simulink model "exampleModel_bus_axi_w_4ptavg"  (R2017b)
settings: Solver=VariableStepAuto  StartTime=0.0  StopTime=10e-5  RelTol=1e-3
PreLoadFcn:
  | setup
values from neighbouring files (symbols this model uses):
  axiClk = 156.25e6    (= 156250000)    [setup.m]    (also in setup_exampleModel_bus_axi_simulink.m; setup_exampleModel_bus_axi_simulink_lcls2.m; setup_lcls2_pcav.m; sysgen_signal.m)
  cav1p1_addr = 204    [setup_exampleModel_bus_axi_simulink.m]    (also in setup_exampleModel_bus_axi_simulink_lcls2.m; setup_lcls2_pcav.m; sysgen_signal.m)
  cav1p2_addr = cav1p1_addr * 2    (= 408)    [setup_exampleModel_bus_axi_simulink.m]    (also in setup_exampleModel_bus_axi_simulink_lcls2.m; setup_lcls2_pcav.m; sysgen_signal.m)
  cav2p1_addr = cav1p1_addr * 3    (= 612)    [setup_exampleModel_bus_axi_simulink.m]    (also in setup_exampleModel_bus_axi_simulink_lcls2.m; setup_lcls2_pcav.m; sysgen_signal.m)
  cav2p2_addr = cav1p1_addr * 4    (= 816)    [setup_exampleModel_bus_axi_simulink.m]    (also in setup_exampleModel_bus_axi_simulink_lcls2.m; setup_lcls2_pcav.m; sysgen_signal.m)
  Fadc = Fs/interleavedChannels    (= 29750000)    [setup.m]    (also in setup_exampleModel_bus_axi_simulink.m = 357000000; setup_exampleModel_bus_axi_simulink_lcls2.m = 351000000; setup_lcls2_pcav.m = 357000000; sysgen_signal.m = 357000000)
  fir_lpf = fir1(15, w_lpf)    [setup_exampleModel_bus_axi_simulink.m]    (also in setup_exampleModel_bus_axi_simulink_lcls2.m; setup_lcls2_pcav.m)
  Fproc = 204e6    (= 204000000)    [setup_exampleModel_bus_axi_simulink.m]    (also in setup_exampleModel_bus_axi_simulink_lcls2.m = 200571400; setup_lcls2_pcav.m; sysgen_signal.m)
  Fsig = Fproc/12    (= 17000000)    [setup_exampleModel_bus_axi_simulink.m]    (also in setup_exampleModel_bus_axi_simulink_lcls2.m = 16714283.3333; setup_lcls2_pcav.m)
  Tadc = 1/fadc    (= 2.80112044818e-09)    [cavity_signal.m]    (also in setup_exampleModel_bus_axi_simulink.m; setup_exampleModel_bus_axi_simulink_lcls2.m = 2.849002849e-09; setup_lcls2_pcav.m; setup_pcav_simulink.m)
undefined symbols (not defined in the file or in its folder): AXI4, Lite
libraries: xbsIndex_r4 x2870, llrf_lib x10, simulink x3
(part 12 of 15)

== system exampleModel_bus_axi_w_4ptavg/example/dsp/Cav2/Subsystem2/freq_err1 ==
  note: window for start/stop evaluating the phase
  note: f=w/(2*pi)
  note: w = d_phi/dt = (pi*(scaled_phi))/dt
  note: pi*(scaled_phi))
  note: 2*pi*dt
  note: find ratio with NCO
  raw_phase : Inport
  window : Inport  Port=2
  reset : Inport  Port=3
  Constant8 : xbsIndex_r4/Constant  const=-Fsig  gui_display_data_type=Fixed-point  arith_type=Signed (2's comp)  n_bits=26  bin_pt=0  preci_type=Single  exp_width=8  frac_width=24  explicit_period=off  period=1  equ=P=C  opselect=C  inp2=PCIN>>17  opr=+  inp1=P  carry=CIN  dbl_ovrd=off  block_type=constant
  Convert : xbsIndex_r4/Convert  gui_display_data_type=Fixed-point  arith_type="Signed  (2's comp)"  n_bits=32  bin_pt=32  float_type=Single  exp_bits=8  fraction_bits=24  quantization=Truncate  overflow=Saturate  en=off  latency=1  pipeline=off  dbl_ovrd=off  block_type=convert
  Convert1 : xbsIndex_r4/Convert  gui_display_data_type=Fixed-point  arith_type="Signed  (2's comp)"  n_bits=32  bin_pt=10  float_type=Single  exp_bits=8  fraction_bits=24  quantization=Truncate  overflow=Saturate  en=off  latency=1  pipeline=off  dbl_ovrd=off  block_type=convert
  Convert3 : xbsIndex_r4/Convert  gui_display_data_type=Boolean  arith_type=Boolean  n_bits=16  bin_pt=14  float_type=Single  exp_bits=8  fraction_bits=24  quantization=Truncate  overflow=Wrap  en=off  latency=1  pipeline=off  dbl_ovrd=off  block_type=convert
  Delay : Delay  DelayLength=3  InitialCondition=0
  Delay1 : Delay  DelayLength=3  InitialCondition=0
  Delay2 : Delay  DelayLength=3  InitialCondition=0
  Display6 : Display
  Display8 : Display
  Divide : xbsIndex_r4/Divide  flow_control=NonBlocking  axi_optimize_goal=Resources  algorithm_type=Radix2  infoedit1=Specify output fraction-width for Fixed-point division.  fractional_width=31  infoedit2=Specify latency for Floating-point division.  latency=1  rate=1  has_a_tlast=off  has_a_tuser=off  has_b_tlast=off  has_b_tuser=off  en=off  has_result_tready=off  result_tlast_behv=Pass_A_TLAST  has_underflow=off  has_overflow=off  has_invalid_op=off  has_divide_by_zero=off  fpo_op_type=mergeddivide  block_type=divide
      settings: infoedit=Blocking: Wait for data on all inputs, allow back-pressure.<br>NonBlocking: operate every cycle in which all inputs are valid, no back-pressure.
  Divide1 : xbsIndex_r4/Divide  flow_control=NonBlocking  axi_optimize_goal=Resources  algorithm_type=Radix2  infoedit1=Specify output fraction-width for Fixed-point division.  fractional_width=33  infoedit2=Specify latency for Floating-point division.  latency=1  rate=1  has_a_tlast=off  has_a_tuser=off  has_b_tlast=off  has_b_tuser=off  en=off  has_result_tready=off  result_tlast_behv=Pass_A_TLAST  has_underflow=off  has_overflow=off  has_invalid_op=off  has_divide_by_zero=off  fpo_op_type=mergeddivide  block_type=divide
      settings: infoedit=Blocking: Wait for data on all inputs, allow back-pressure.<br>NonBlocking: operate every cycle in which all inputs are valid, no back-pressure.
  Down Sample : xbsIndex_r4/Down Sample  sample_ratio=12  sample_phase="Last Value of Frame  (most efficient)"  en=off  rst=off  latency=1  dbl_ovrd=off  block_type=dsamp
  Gateway Out{1..5,11,19..20} (8 alike) : xbsIndex_r4/Gateway Out  inherit_from_input=off  hdl_port=on  rows=1  columns=1  UseAsDAC=off  DACChannel='1'  interface=None  automatic_assignment=on  address_offset=hex2dec('00')  intf_name=''  intf_description=''  timing_constraint=None  locs_specified=off  LOCs={}  io_standard={}  block_type=gatewayout
  Mult3 : xbsIndex_r4/Mult  precision=User Defined  arith_type="Signed  (2's comp)"  n_bits=18  bin_pt=15  quantization=Truncate  overflow=Saturate  en=off  latency=3  use_behavioral_HDL=off  opt=Speed  use_embedded=on  optimum_pipeline=off  pipeline=on  dbl_ovrd=off  use_rpm=on  placement_style=Triangular  block_type=mult
  Scope1 : Scope  NumInputPorts=2
  Scope2 : Scope  NumInputPorts=3
  Subsystem : Subsystem  Commented=on
  delta_phi : Subsystem
  delta_t : Subsystem
  lo_bit_phi : Scope  NumInputPorts=4
  NCO_err : Outport
  freq_err : Outport  Port=2
  wires:
  Divide/1 -> Subsystem/2(In2), Divide1/1, Convert1/1
  Convert/1 -> Gateway Out11/1, NCO_err/1
  Delay1/1 -> lo_bit_phi/1, Scope2/3
  raw_phase/1 -> Gateway Out3/1, Mult3/2, Gateway Out1/1, Gateway Out2/1
  Delay2/1 -> lo_bit_phi/4
  Gateway Out4/1 -> Delay2/1
  [c1p2_pt_cntr] -> Gateway Out4/1
  Delay/1 -> lo_bit_phi/3
  Gateway Out3/1 -> Delay/1
  Gateway Out2/1 -> Scope1/1
  Gateway Out1/1 -> Scope1/2
  Divide1/1 -> Down Sample/1
  Down Sample/1 -> Convert/1
  Constant8/1 -> Divide1/2
  Mult3/1 -> Gateway Out19/1, delta_phi/1(phase)
  window/1 -> Mult3/1, delta_phi/2(window), delta_t/1(window), Gateway Out20/1
  Gateway Out19/1 -> lo_bit_phi/2
  Convert3/1 -> delta_phi/3(reset), delta_t/2(reset)
  Gateway Out20/1 -> Delay1/1
  Gateway Out5/1 -> Scope2/1, Display6/1
  Gateway Out11/1 -> Display8/1, Scope2/2
  reset/1 -> Convert3/1
  delta_phi/1(d_phi) -> Divide/1
  delta_t/1(dt) -> Divide/2
  delta_phi/2(val_latched) -> Subsystem/1(In1)
  Convert1/1 -> freq_err/1, Gateway Out5/1

== system exampleModel_bus_axi_w_4ptavg/example/dsp/Cav2/Subsystem4/four_point_avg1 ==
  In1 : Inport
  AddSub1 : xbsIndex_r4/AddSub  mode=Addition  use_carryin=off  use_carryout=off  en=off  latency=1  precision=User Defined  arith_type="Signed  (2's comp)"  n_bits=33  bin_pt=31  quantization=Truncate  overflow=Saturate  use_behavioral_HDL=off  hw_selection=Fabric  pipelined=off  dbl_ovrd=off  block_type=addsub
  AddSub2 : xbsIndex_r4/AddSub  mode=Addition  use_carryin=off  use_carryout=off  en=off  latency=1  precision=User Defined  arith_type="Signed  (2's comp)"  n_bits=33  bin_pt=31  quantization=Truncate  overflow=Saturate  use_behavioral_HDL=off  hw_selection=Fabric  pipelined=off  dbl_ovrd=off  block_type=addsub
  AddSub3 : xbsIndex_r4/AddSub  mode=Addition  use_carryin=off  use_carryout=off  en=off  latency=1  precision=User Defined  arith_type="Signed  (2's comp)"  n_bits=33  bin_pt=31  quantization=Truncate  overflow=Saturate  use_behavioral_HDL=off  hw_selection=Fabric  pipelined=off  dbl_ovrd=off  block_type=addsub
  CMult{1..4} (4 alike) : xbsIndex_r4/CMult  const=0.25  gui_display_data_type=Fixed-point  const_n_bits=18  const_bin_pt=16  float_type=Single  exp_bits=8  fraction_bits=24  en=off  latency=1  precision=User Defined  arith_type="Signed  (2's comp)"  n_bits=33  bin_pt=31  quantization=Truncate  overflow=Saturate  use_behavioral_HDL=off  mem_type=Distributed RAM  pipeline=off  dbl_ovrd=off  block_type=cmult
  Delay1 : xbsIndex_r4/Delay  rst=off  infoeditControl=Selection of Reset will increase slice count due to use of real FFs and instead of SRLs  en=off  latency=1  reg_retiming=off  dbl_ovrd=off  block_type=delay
  Delay2 : xbsIndex_r4/Delay  rst=off  infoeditControl=Selection of Reset will increase slice count due to use of real FFs and instead of SRLs  en=off  latency=1  reg_retiming=off  dbl_ovrd=off  block_type=delay
  Delay3 : xbsIndex_r4/Delay  rst=off  infoeditControl=Selection of Reset will increase slice count due to use of real FFs and instead of SRLs  en=off  latency=1  reg_retiming=off  dbl_ovrd=off  block_type=delay
  Out1 : Outport
  wires:
  CMult1/1 -> AddSub2/1
  CMult4/1 -> AddSub1/1
  AddSub3/1 -> Out1/1
  CMult3/1 -> AddSub2/2
  In1/1 -> Delay1/1, CMult4/1
  AddSub1/1 -> AddSub3/2
  Delay3/1 -> CMult3/1
  CMult2/1 -> AddSub1/2
  Delay2/1 -> Delay3/1, CMult1/1
  AddSub2/1 -> AddSub3/1
  Delay1/1 -> Delay2/1, CMult2/1

== system exampleModel_bus_axi_w_4ptavg/example/dsp/Cav2/Subsystem4/freq_err1 ==
  note: window for start/stop evaluating the phase
  note: f=w/(2*pi)
  note: w = d_phi/dt = (pi*(scaled_phi))/dt
  note: pi*(scaled_phi))
  note: 2*pi*dt
  note: find ratio with NCO
  raw_phase : Inport
  window : Inport  Port=2
  reset : Inport  Port=3
  Constant8 : xbsIndex_r4/Constant  const=-Fsig  gui_display_data_type=Fixed-point  arith_type=Signed (2's comp)  n_bits=26  bin_pt=0  preci_type=Single  exp_width=8  frac_width=24  explicit_period=off  period=1  equ=P=C  opselect=C  inp2=PCIN>>17  opr=+  inp1=P  carry=CIN  dbl_ovrd=off  block_type=constant
  Convert : xbsIndex_r4/Convert  gui_display_data_type=Fixed-point  arith_type="Signed  (2's comp)"  n_bits=32  bin_pt=32  float_type=Single  exp_bits=8  fraction_bits=24  quantization=Truncate  overflow=Saturate  en=off  latency=1  pipeline=off  dbl_ovrd=off  block_type=convert
  Convert1 : xbsIndex_r4/Convert  gui_display_data_type=Fixed-point  arith_type="Signed  (2's comp)"  n_bits=32  bin_pt=10  float_type=Single  exp_bits=8  fraction_bits=24  quantization=Truncate  overflow=Saturate  en=off  latency=1  pipeline=off  dbl_ovrd=off  block_type=convert
  Convert3 : xbsIndex_r4/Convert  gui_display_data_type=Boolean  arith_type=Boolean  n_bits=16  bin_pt=14  float_type=Single  exp_bits=8  fraction_bits=24  quantization=Truncate  overflow=Wrap  en=off  latency=1  pipeline=off  dbl_ovrd=off  block_type=convert
  Delay : Delay  DelayLength=3  InitialCondition=0
  Delay1 : Delay  DelayLength=3  InitialCondition=0
  Delay2 : Delay  DelayLength=3  InitialCondition=0
  Delay3 : xbsIndex_r4/Delay  rst=off  infoeditControl=Selection of Reset will increase slice count due to use of real FFs and instead of SRLs  en=off  latency=4  reg_retiming=off  dbl_ovrd=off  block_type=delay
  Display6 : Display
  Display8 : Display
  Divide : xbsIndex_r4/Divide  flow_control=NonBlocking  axi_optimize_goal=Resources  algorithm_type=Radix2  infoedit1=Specify output fraction-width for Fixed-point division.  fractional_width=31  infoedit2=Specify latency for Floating-point division.  latency=1  rate=1  has_a_tlast=off  has_a_tuser=off  has_b_tlast=off  has_b_tuser=off  en=off  has_result_tready=off  result_tlast_behv=Pass_A_TLAST  has_underflow=off  has_overflow=off  has_invalid_op=off  has_divide_by_zero=off  fpo_op_type=mergeddivide  block_type=divide
      settings: infoedit=Blocking: Wait for data on all inputs, allow back-pressure.<br>NonBlocking: operate every cycle in which all inputs are valid, no back-pressure.
  Divide1 : xbsIndex_r4/Divide  flow_control=NonBlocking  axi_optimize_goal=Resources  algorithm_type=Radix2  infoedit1=Specify output fraction-width for Fixed-point division.  fractional_width=33  infoedit2=Specify latency for Floating-point division.  latency=1  rate=1  has_a_tlast=off  has_a_tuser=off  has_b_tlast=off  has_b_tuser=off  en=off  has_result_tready=off  result_tlast_behv=Pass_A_TLAST  has_underflow=off  has_overflow=off  has_invalid_op=off  has_divide_by_zero=off  fpo_op_type=mergeddivide  block_type=divide
      settings: infoedit=Blocking: Wait for data on all inputs, allow back-pressure.<br>NonBlocking: operate every cycle in which all inputs are valid, no back-pressure.
  Down Sample : xbsIndex_r4/Down Sample  sample_ratio=12  sample_phase="Last Value of Frame  (most efficient)"  en=off  rst=off  latency=1  dbl_ovrd=off  block_type=dsamp
  Gateway Out{1..6,11,19..20} (9 alike) : xbsIndex_r4/Gateway Out  inherit_from_input=off  hdl_port=on  rows=1  columns=1  UseAsDAC=off  DACChannel='1'  interface=None  automatic_assignment=on  address_offset=hex2dec('00')  intf_name=''  intf_description=''  timing_constraint=None  locs_specified=off  LOCs={}  io_standard={}  block_type=gatewayout
  Inverter : xbsIndex_r4/Inverter  en=off  latency=1  dbl_ovrd=off  block_type=inv
  Logical : xbsIndex_r4/Logical  logical_function=AND  inputs=2  en=off  latency=1  precision=Full  arith_type=Unsigned  n_bits=16  bin_pt=0  align_bp=on  dbl_ovrd=off  block_type=logical
  Mult3 : xbsIndex_r4/Mult  precision=User Defined  arith_type="Signed  (2's comp)"  n_bits=18  bin_pt=15  quantization=Truncate  overflow=Saturate  en=off  latency=3  use_behavioral_HDL=off  opt=Speed  use_embedded=on  optimum_pipeline=off  pipeline=on  dbl_ovrd=off  use_rpm=on  placement_style=Triangular  block_type=mult
  Scope1 : Scope  NumInputPorts=2
  Scope2 : Scope  NumInputPorts=3
  Scope3 : Scope  NumInputPorts=2
  Subsystem : Subsystem  Commented=on
  delta_phi : Subsystem
  delta_t : Subsystem
  lo_bit_phi : Scope  NumInputPorts=4
  NCO_err : Outport
  freq_err : Outport  Port=2
  wires:
  Divide/1 -> Subsystem/2(In2), Divide1/1, Convert1/1
  Convert/1 -> Gateway Out11/1, NCO_err/1
  Delay1/1 -> lo_bit_phi/1, Scope2/3
  raw_phase/1 -> Gateway Out3/1, Mult3/2, Gateway Out1/1, Gateway Out2/1
  Delay2/1 -> lo_bit_phi/4
  Gateway Out4/1 -> Delay2/1
  [c1p2_pt_cntr] -> Gateway Out4/1
  Delay/1 -> lo_bit_phi/3
  Gateway Out3/1 -> Delay/1
  Gateway Out2/1 -> Scope1/1
  Gateway Out1/1 -> Scope1/2
  Divide1/1 -> Down Sample/1
  Down Sample/1 -> Convert/1
  Constant8/1 -> Divide1/2
  Mult3/1 -> Gateway Out19/1, delta_phi/1(phase)
  window/1 -> Mult3/1, delta_phi/2(window), delta_t/1(window), Delay3/1, Inverter/1, Gateway Out20/1
  Gateway Out19/1 -> lo_bit_phi/2
  Convert3/1 -> delta_phi/3(reset), delta_t/2(reset)
  Gateway Out20/1 -> Scope3/2, Delay1/1
  Gateway Out5/1 -> Scope2/1, Display6/1
  Gateway Out11/1 -> Display8/1, Scope2/2
  reset/1 -> Convert3/1
  delta_phi/1(d_phi) -> Divide/1
  delta_t/1(dt) -> Divide/2
  delta_phi/2(val_latched) -> Subsystem/1(In1)
  Convert1/1 -> freq_err/1, Gateway Out5/1
  Inverter/1 -> Logical/1
  Delay3/1 -> Logical/2
  Logical/1 -> Gateway Out6/1
  Gateway Out6/1 -> Scope3/1

== system exampleModel_bus_axi_w_4ptavg/example/dsp/Cav2/Subsystem5/posedge_pulse ==
  In1 : Inport
  Inverter1 : xbsIndex_r4/Inverter  en=off  latency=1  dbl_ovrd=off  block_type=inv
  Logical : xbsIndex_r4/Logical  logical_function=AND  inputs=2  en=off  latency=1  precision=Full  arith_type=Unsigned  n_bits=16  bin_pt=0  align_bp=on  dbl_ovrd=off  block_type=logical
  Out1 : Outport
  wires:
  Inverter1/1 -> Logical/2
  Logical/1 -> Out1/1
  In1/1 -> Inverter1/1, Logical/1

== system exampleModel_bus_axi_w_4ptavg/example/dsp/Cav2/Subsystem6/posedge_pulse ==
  In1 : Inport
  Inverter1 : xbsIndex_r4/Inverter  en=off  latency=1  dbl_ovrd=off  block_type=inv
  Logical : xbsIndex_r4/Logical  logical_function=AND  inputs=2  en=off  latency=1  precision=Full  arith_type=Unsigned  n_bits=16  bin_pt=0  align_bp=on  dbl_ovrd=off  block_type=logical
  Out1 : Outport
  wires:
  In1/1 -> Logical/1, Inverter1/1
  Logical/1 -> Out1/1
  Inverter1/1 -> Logical/2

== system exampleModel_bus_axi_w_4ptavg/example/dsp/Cav2/Subsystem7/posedge_pulse ==
  In1 : Inport
  Inverter1 : xbsIndex_r4/Inverter  en=off  latency=1  dbl_ovrd=off  block_type=inv
  Logical : xbsIndex_r4/Logical  logical_function=AND  inputs=2  en=off  latency=1  precision=Full  arith_type=Unsigned  n_bits=16  bin_pt=0  align_bp=on  dbl_ovrd=off  block_type=logical
  Out1 : Outport
  wires:
  Inverter1/1 -> Logical/2
  Logical/1 -> Out1/1
  In1/1 -> Inverter1/1, Logical/1

== system exampleModel_bus_axi_w_4ptavg/example/dsp/Cav2/Subsystem8/posedge_pulse ==
  In1 : Inport
  Inverter1 : xbsIndex_r4/Inverter  en=off  latency=1  dbl_ovrd=off  block_type=inv
  Logical : xbsIndex_r4/Logical  logical_function=AND  inputs=2  en=off  latency=1  precision=Full  arith_type=Unsigned  n_bits=16  bin_pt=0  align_bp=on  dbl_ovrd=off  block_type=logical
  Out1 : Outport
  wires:
  In1/1 -> Logical/1, Inverter1/1
  Logical/1 -> Out1/1
  Inverter1/1 -> Logical/2

== system exampleModel_bus_axi_w_4ptavg/example/dsp/Cav2/Subsystem9/posedge_pulse ==
  In1 : Inport
  Inverter1 : xbsIndex_r4/Inverter  en=off  latency=1  dbl_ovrd=off  block_type=inv
  Logical : xbsIndex_r4/Logical  logical_function=AND  inputs=2  en=off  latency=1  precision=Full  arith_type=Unsigned  n_bits=16  bin_pt=0  align_bp=on  dbl_ovrd=off  block_type=logical
  Out1 : Outport
  wires:
  Inverter1/1 -> Logical/2
  Logical/1 -> Out1/1
  In1/1 -> Inverter1/1, Logical/1

== system exampleModel_bus_axi_w_4ptavg/example/dsp/Cav2/c1p2_windowing_func2/four_point_avg ==
  In1 : Inport
  AddSub1 : xbsIndex_r4/AddSub  mode=Addition  use_carryin=off  use_carryout=off  en=off  latency=1  precision=User Defined  arith_type="Signed  (2's comp)"  n_bits=18  bin_pt=15  quantization=Truncate  overflow=Saturate  use_behavioral_HDL=off  hw_selection=Fabric  pipelined=off  dbl_ovrd=off  block_type=addsub
  AddSub2 : xbsIndex_r4/AddSub  mode=Addition  use_carryin=off  use_carryout=off  en=off  latency=1  precision=User Defined  arith_type="Signed  (2's comp)"  n_bits=18  bin_pt=15  quantization=Truncate  overflow=Saturate  use_behavioral_HDL=off  hw_selection=Fabric  pipelined=off  dbl_ovrd=off  block_type=addsub
  AddSub3 : xbsIndex_r4/AddSub  mode=Addition  use_carryin=off  use_carryout=off  en=off  latency=1  precision=User Defined  arith_type="Signed  (2's comp)"  n_bits=18  bin_pt=15  quantization=Truncate  overflow=Saturate  use_behavioral_HDL=off  hw_selection=Fabric  pipelined=off  dbl_ovrd=off  block_type=addsub
  CMult{1..4} (4 alike) : xbsIndex_r4/CMult  const=0.25  gui_display_data_type=Fixed-point  const_n_bits=18  const_bin_pt=16  float_type=Single  exp_bits=8  fraction_bits=24  en=off  latency=1  precision=User Defined  arith_type="Signed  (2's comp)"  n_bits=18  bin_pt=16  quantization=Truncate  overflow=Saturate  use_behavioral_HDL=off  mem_type=Distributed RAM  pipeline=off  dbl_ovrd=off  block_type=cmult
  Delay1 : xbsIndex_r4/Delay  rst=off  infoeditControl=Selection of Reset will increase slice count due to use of real FFs and instead of SRLs  en=off  latency=1  reg_retiming=off  dbl_ovrd=off  block_type=delay
  Delay2 : xbsIndex_r4/Delay  rst=off  infoeditControl=Selection of Reset will increase slice count due to use of real FFs and instead of SRLs  en=off  latency=1  reg_retiming=off  dbl_ovrd=off  block_type=delay
  Delay3 : xbsIndex_r4/Delay  rst=off  infoeditControl=Selection of Reset will increase slice count due to use of real FFs and instead of SRLs  en=off  latency=1  reg_retiming=off  dbl_ovrd=off  block_type=delay
  Out1 : Outport
  wires:
  CMult1/1 -> AddSub2/1
  CMult4/1 -> AddSub1/1
  AddSub3/1 -> Out1/1
  CMult3/1 -> AddSub2/2
  In1/1 -> CMult4/1, Delay1/1
  AddSub1/1 -> AddSub3/2
  Delay3/1 -> CMult3/1
  CMult2/1 -> AddSub1/2
  Delay2/1 -> CMult1/1, Delay3/1
  AddSub2/1 -> AddSub3/1
  Delay1/1 -> CMult2/1, Delay2/1

== system exampleModel_bus_axi_w_4ptavg/example/dsp/Cav2/c1p2_windowing_func3/four_point_avg ==
  In1 : Inport
  AddSub1 : xbsIndex_r4/AddSub  mode=Addition  use_carryin=off  use_carryout=off  en=off  latency=1  precision=User Defined  arith_type="Signed  (2's comp)"  n_bits=18  bin_pt=15  quantization=Truncate  overflow=Saturate  use_behavioral_HDL=off  hw_selection=Fabric  pipelined=off  dbl_ovrd=off  block_type=addsub
  AddSub2 : xbsIndex_r4/AddSub  mode=Addition  use_carryin=off  use_carryout=off  en=off  latency=1  precision=User Defined  arith_type="Signed  (2's comp)"  n_bits=18  bin_pt=15  quantization=Truncate  overflow=Saturate  use_behavioral_HDL=off  hw_selection=Fabric  pipelined=off  dbl_ovrd=off  block_type=addsub
  AddSub3 : xbsIndex_r4/AddSub  mode=Addition  use_carryin=off  use_carryout=off  en=off  latency=1  precision=User Defined  arith_type="Signed  (2's comp)"  n_bits=18  bin_pt=15  quantization=Truncate  overflow=Saturate  use_behavioral_HDL=off  hw_selection=Fabric  pipelined=off  dbl_ovrd=off  block_type=addsub
  CMult{1..4} (4 alike) : xbsIndex_r4/CMult  const=0.25  gui_display_data_type=Fixed-point  const_n_bits=18  const_bin_pt=16  float_type=Single  exp_bits=8  fraction_bits=24  en=off  latency=1  precision=User Defined  arith_type="Signed  (2's comp)"  n_bits=18  bin_pt=16  quantization=Truncate  overflow=Saturate  use_behavioral_HDL=off  mem_type=Distributed RAM  pipeline=off  dbl_ovrd=off  block_type=cmult
  Delay1 : xbsIndex_r4/Delay  rst=off  infoeditControl=Selection of Reset will increase slice count due to use of real FFs and instead of SRLs  en=off  latency=1  reg_retiming=off  dbl_ovrd=off  block_type=delay
  Delay2 : xbsIndex_r4/Delay  rst=off  infoeditControl=Selection of Reset will increase slice count due to use of real FFs and instead of SRLs  en=off  latency=1  reg_retiming=off  dbl_ovrd=off  block_type=delay
  Delay3 : xbsIndex_r4/Delay  rst=off  infoeditControl=Selection of Reset will increase slice count due to use of real FFs and instead of SRLs  en=off  latency=1  reg_retiming=off  dbl_ovrd=off  block_type=delay
  Out1 : Outport
  wires:
  Delay1/1 -> Delay2/1, CMult2/1
  AddSub2/1 -> AddSub3/1
  Delay2/1 -> Delay3/1, CMult1/1
  CMult2/1 -> AddSub1/2
  Delay3/1 -> CMult3/1
  AddSub1/1 -> AddSub3/2
  In1/1 -> Delay1/1, CMult4/1
  CMult3/1 -> AddSub2/2
  AddSub3/1 -> Out1/1
  CMult4/1 -> AddSub1/1
  CMult1/1 -> AddSub2/1

== system exampleModel_bus_axi_w_4ptavg/example/dsp/Cav2/c2p1_window_wf /Delay_calc1 ==
  wav : Inport
  win : Inport  Port=2
  Absolute1 : xbsIndex_r4/Absolute  precision=Full  arith_type=Unsigned  n_bits=16  bin_pt=14  quantization=Truncate  overflow=Wrap  en=off  latency=1  dbl_ovrd=off  block_type=abs
  Absolute2 : xbsIndex_r4/Absolute  precision=Full  arith_type=Unsigned  n_bits=16  bin_pt=14  quantization=Truncate  overflow=Wrap  en=off  latency=1  dbl_ovrd=off  block_type=abs
  Constant1 : xbsIndex_r4/Constant  const=0  gui_display_data_type=Fixed-point  arith_type=Signed (2's comp)  n_bits=18  bin_pt=16  preci_type=Single  exp_width=8  frac_width=24  explicit_period=off  period=1  equ=P=C  opselect=C  inp2=PCIN>>17  opr=+  inp1=P  carry=CIN  dbl_ovrd=off  block_type=constant
  Constant2 : xbsIndex_r4/Constant  const=0  gui_display_data_type=Fixed-point  arith_type=Signed (2's comp)  n_bits=2  bin_pt=0  preci_type=Single  exp_width=8  frac_width=24  explicit_period=off  period=1  equ=P=C  opselect=C  inp2=PCIN>>17  opr=+  inp1=P  carry=CIN  dbl_ovrd=off  block_type=constant
  Counter : xbsIndex_r4/Counter  cnt_type=Free Running  cnt_to=Inf  operation=Up  start_count=0  cnt_by_val=1  arith_type=Unsigned  n_bits=16  bin_pt=0  load_pin=off  rst=on  en=on  explicit_period=off  period=1  use_behavioral_HDL=off  implementation=Fabric  dbl_ovrd=off  block_type=counter
  Delay2 : xbsIndex_r4/Delay  rst=off  infoeditControl=Selection of Reset will increase slice count due to use of real FFs and instead of SRLs  en=off  latency=30  reg_retiming=off  dbl_ovrd=off  block_type=delay
  Display : Display
  Gateway Out{1..11,18..19} (13 alike) : xbsIndex_r4/Gateway Out  inherit_from_input=off  hdl_port=off  rows=1  columns=1  UseAsDAC=off  DACChannel='1'  interface=None  automatic_assignment=on  address_offset=hex2dec('00')  intf_name=''  intf_description=''  timing_constraint=None  locs_specified=off  LOCs={}  io_standard={}  block_type=gatewayout
  Logical3 : xbsIndex_r4/Logical  logical_function=XOR  inputs=2  en=off  latency=1  precision=Full  arith_type=Unsigned  n_bits=16  bin_pt=0  align_bp=on  dbl_ovrd=off  block_type=logical
  Register2 : xbsIndex_r4/Register  init=0  rst=off  en=on  dbl_ovrd=off  block_type=register
  Relational1 : xbsIndex_r4/Relational  mode=a>b  op_type=Bool  en=off  latency=1  dbl_ovrd=off  block_type=relational
  Relational3 : xbsIndex_r4/Relational  mode=a>b  op_type=Bool  en=off  latency=1  dbl_ovrd=off  block_type=relational
  Scope{1..2,4,7} (4 alike) : Scope  NumInputPorts=3
  Scope3 : Scope  NumInputPorts=2
  Subsystem : Subsystem
  Subsystem1 : Subsystem
  Subsystem2 : Subsystem
  Subsystem3 : Subsystem
  negedge : Subsystem
  delay_amt : Outport
  delay_fb_latch : Outport  Port=2
  wires:
  Register2/1 -> Gateway Out4/1, Gateway Out6/1, delay_amt/1
  Gateway Out19/1 -> Scope3/2
  Constant2/1 -> Relational3/2
  win/1 -> Absolute2/1
  Constant1/1 -> Relational1/2
  Gateway Out18/1 -> Scope3/1
  wav/1 -> Absolute1/1
  Gateway Out6/1 -> Display/1, Scope7/3
  Gateway Out8/1 -> Scope7/2
  Gateway Out7/1 -> Scope7/1
  Gateway Out3/1 -> Scope2/1
  Gateway Out4/1 -> Scope2/2
  Gateway Out5/1 -> Scope2/3, Scope4/1
  Relational1/1 -> Subsystem3/1(In1), Subsystem2/2(d)
  Absolute1/1 -> Relational1/1, Gateway Out18/1
  Absolute2/1 -> Gateway Out19/1, Relational3/1
  Gateway Out9/1 -> Scope4/3
  Gateway Out10/1 -> Scope4/2
  Counter/1 -> Register2/1, Gateway Out8/1, Gateway Out5/1
  Logical3/1 -> Gateway Out11/1, Gateway Out10/1, Counter/2
  [reset] -> Gateway Out9/1, Counter/1
  Delay2/1 -> Gateway Out3/1, delay_fb_latch/1
  Relational3/1 -> Subsystem1/2(d), Subsystem/1(In1), Subsystem3/2(In2)
  negedge/1(q) -> Register2/2, Subsystem2/1(lc), Subsystem1/1(lc)
  Subsystem1/1(q) -> Subsystem1/3(qb), Gateway Out2/1, Logical3/2
  Subsystem2/1(q) -> Subsystem2/3(qb), Gateway Out1/1, Logical3/1
  Subsystem3/2(or) -> negedge/1(d)
  Subsystem3/1(and) -> Gateway Out7/1
  Subsystem/1(Out1) -> Delay2/1
  Gateway Out1/1 -> Scope1/2
  Gateway Out2/1 -> Scope1/3
  Gateway Out11/1 -> Scope1/1

== system exampleModel_bus_axi_w_4ptavg/example/dsp/Cav2/c2p1_window_wf /Delay_calc2 ==
  wav : Inport
  win : Inport  Port=2
  Absolute1 : xbsIndex_r4/Absolute  precision=Full  arith_type=Unsigned  n_bits=16  bin_pt=14  quantization=Truncate  overflow=Wrap  en=off  latency=1  dbl_ovrd=off  block_type=abs
  Absolute2 : xbsIndex_r4/Absolute  precision=Full  arith_type=Unsigned  n_bits=16  bin_pt=14  quantization=Truncate  overflow=Wrap  en=off  latency=1  dbl_ovrd=off  block_type=abs
  Constant1 : xbsIndex_r4/Constant  const=0  gui_display_data_type=Fixed-point  arith_type=Signed (2's comp)  n_bits=18  bin_pt=16  preci_type=Single  exp_width=8  frac_width=24  explicit_period=off  period=1  equ=P=C  opselect=C  inp2=PCIN>>17  opr=+  inp1=P  carry=CIN  dbl_ovrd=off  block_type=constant
  Constant2 : xbsIndex_r4/Constant  const=0  gui_display_data_type=Fixed-point  arith_type=Signed (2's comp)  n_bits=2  bin_pt=0  preci_type=Single  exp_width=8  frac_width=24  explicit_period=off  period=1  equ=P=C  opselect=C  inp2=PCIN>>17  opr=+  inp1=P  carry=CIN  dbl_ovrd=off  block_type=constant
  Counter : xbsIndex_r4/Counter  cnt_type=Free Running  cnt_to=Inf  operation=Up  start_count=0  cnt_by_val=1  arith_type=Unsigned  n_bits=16  bin_pt=0  load_pin=off  rst=on  en=on  explicit_period=off  period=1  use_behavioral_HDL=off  implementation=Fabric  dbl_ovrd=off  block_type=counter
  Delay2 : xbsIndex_r4/Delay  rst=off  infoeditControl=Selection of Reset will increase slice count due to use of real FFs and instead of SRLs  en=off  latency=30  reg_retiming=off  dbl_ovrd=off  block_type=delay
  Display : Display
  Gateway Out{1..11,18..19} (13 alike) : xbsIndex_r4/Gateway Out  inherit_from_input=off  hdl_port=off  rows=1  columns=1  UseAsDAC=off  DACChannel='1'  interface=None  automatic_assignment=on  address_offset=hex2dec('00')  intf_name=''  intf_description=''  timing_constraint=None  locs_specified=off  LOCs={}  io_standard={}  block_type=gatewayout
  Logical3 : xbsIndex_r4/Logical  logical_function=XOR  inputs=2  en=off  latency=1  precision=Full  arith_type=Unsigned  n_bits=16  bin_pt=0  align_bp=on  dbl_ovrd=off  block_type=logical
  Register2 : xbsIndex_r4/Register  init=0  rst=off  en=on  dbl_ovrd=off  block_type=register
  Relational1 : xbsIndex_r4/Relational  mode=a>b  op_type=Bool  en=off  latency=1  dbl_ovrd=off  block_type=relational
  Relational3 : xbsIndex_r4/Relational  mode=a>b  op_type=Bool  en=off  latency=1  dbl_ovrd=off  block_type=relational
  Scope{1..2,4,7} (4 alike) : Scope  NumInputPorts=3
  Scope3 : Scope  NumInputPorts=2
  Subsystem : Subsystem
  Subsystem1 : Subsystem
  Subsystem2 : Subsystem
  Subsystem3 : Subsystem
  negedge : Subsystem
  delay_amt : Outport
  delay_fb_latch : Outport  Port=2
  wires:
  Register2/1 -> Gateway Out4/1, Gateway Out6/1, delay_amt/1
  Gateway Out19/1 -> Scope3/2
  Constant2/1 -> Relational3/2
  win/1 -> Absolute2/1
  Constant1/1 -> Relational1/2
  Gateway Out18/1 -> Scope3/1
  wav/1 -> Absolute1/1
  Gateway Out6/1 -> Display/1, Scope7/3
  Gateway Out8/1 -> Scope7/2
  Gateway Out7/1 -> Scope7/1
  Gateway Out3/1 -> Scope2/1
  Gateway Out4/1 -> Scope2/2
  Gateway Out5/1 -> Scope2/3, Scope4/1
  Relational1/1 -> Subsystem3/1(In1), Subsystem2/2(d)
  Absolute1/1 -> Relational1/1, Gateway Out18/1
  Absolute2/1 -> Gateway Out19/1, Relational3/1
  Gateway Out9/1 -> Scope4/3
  Gateway Out10/1 -> Scope4/2
  Counter/1 -> Register2/1, Gateway Out8/1, Gateway Out5/1
  Logical3/1 -> Gateway Out11/1, Gateway Out10/1, Counter/2
  [reset] -> Gateway Out9/1, Counter/1
  Delay2/1 -> Gateway Out3/1, delay_fb_latch/1
  Relational3/1 -> Subsystem1/2(d), Subsystem/1(In1), Subsystem3/2(In2)
  negedge/1(q) -> Register2/2, Subsystem2/1(lc), Subsystem1/1(lc)
  Subsystem1/1(q) -> Subsystem1/3(qb), Gateway Out2/1, Logical3/2
  Subsystem2/1(q) -> Subsystem2/3(qb), Gateway Out1/1, Logical3/1
  Subsystem3/2(or) -> negedge/1(d)
  Subsystem3/1(and) -> Gateway Out7/1
  Subsystem/1(Out1) -> Delay2/1
  Gateway Out1/1 -> Scope1/2
  Gateway Out2/1 -> Scope1/3
  Gateway Out11/1 -> Scope1/1

== system exampleModel_bus_axi_w_4ptavg/example/dsp/Cav2/c2p2_window_wf/Delay_calc1 ==
  wav : Inport
  win : Inport  Port=2
  Absolute1 : xbsIndex_r4/Absolute  precision=Full  arith_type=Unsigned  n_bits=16  bin_pt=14  quantization=Truncate  overflow=Wrap  en=off  latency=1  dbl_ovrd=off  block_type=abs
  Absolute2 : xbsIndex_r4/Absolute  precision=Full  arith_type=Unsigned  n_bits=16  bin_pt=14  quantization=Truncate  overflow=Wrap  en=off  latency=1  dbl_ovrd=off  block_type=abs
  Constant1 : xbsIndex_r4/Constant  const=0  gui_display_data_type=Fixed-point  arith_type=Signed (2's comp)  n_bits=18  bin_pt=16  preci_type=Single  exp_width=8  frac_width=24  explicit_period=off  period=1  equ=P=C  opselect=C  inp2=PCIN>>17  opr=+  inp1=P  carry=CIN  dbl_ovrd=off  block_type=constant
  Constant2 : xbsIndex_r4/Constant  const=0  gui_display_data_type=Fixed-point  arith_type=Signed (2's comp)  n_bits=2  bin_pt=0  preci_type=Single  exp_width=8  frac_width=24  explicit_period=off  period=1  equ=P=C  opselect=C  inp2=PCIN>>17  opr=+  inp1=P  carry=CIN  dbl_ovrd=off  block_type=constant
  Counter : xbsIndex_r4/Counter  cnt_type=Free Running  cnt_to=Inf  operation=Up  start_count=0  cnt_by_val=1  arith_type=Unsigned  n_bits=16  bin_pt=0  load_pin=off  rst=on  en=on  explicit_period=off  period=1  use_behavioral_HDL=off  implementation=Fabric  dbl_ovrd=off  block_type=counter
  Delay2 : xbsIndex_r4/Delay  rst=off  infoeditControl=Selection of Reset will increase slice count due to use of real FFs and instead of SRLs  en=off  latency=30  reg_retiming=off  dbl_ovrd=off  block_type=delay
  Display : Display
  Gateway Out{1..11,18..19} (13 alike) : xbsIndex_r4/Gateway Out  inherit_from_input=off  hdl_port=off  rows=1  columns=1  UseAsDAC=off  DACChannel='1'  interface=None  automatic_assignment=on  address_offset=hex2dec('00')  intf_name=''  intf_description=''  timing_constraint=None  locs_specified=off  LOCs={}  io_standard={}  block_type=gatewayout
  Logical3 : xbsIndex_r4/Logical  logical_function=XOR  inputs=2  en=off  latency=1  precision=Full  arith_type=Unsigned  n_bits=16  bin_pt=0  align_bp=on  dbl_ovrd=off  block_type=logical
  Register2 : xbsIndex_r4/Register  init=0  rst=off  en=on  dbl_ovrd=off  block_type=register
  Relational1 : xbsIndex_r4/Relational  mode=a>b  op_type=Bool  en=off  latency=1  dbl_ovrd=off  block_type=relational
  Relational3 : xbsIndex_r4/Relational  mode=a>b  op_type=Bool  en=off  latency=1  dbl_ovrd=off  block_type=relational
  Scope{1..2,4,7} (4 alike) : Scope  NumInputPorts=3
  Scope3 : Scope  NumInputPorts=2
  Subsystem : Subsystem
  Subsystem1 : Subsystem
  Subsystem2 : Subsystem
  Subsystem3 : Subsystem
  negedge : Subsystem
  delay_amt : Outport
  delay_fb_latch : Outport  Port=2
  wires:
  Register2/1 -> Gateway Out4/1, Gateway Out6/1, delay_amt/1
  Gateway Out19/1 -> Scope3/2
  Constant2/1 -> Relational3/2
  win/1 -> Absolute2/1
  Constant1/1 -> Relational1/2
  Gateway Out18/1 -> Scope3/1
  wav/1 -> Absolute1/1
  Gateway Out6/1 -> Display/1, Scope7/3
  Gateway Out8/1 -> Scope7/2
  Gateway Out7/1 -> Scope7/1
  Gateway Out3/1 -> Scope2/1
  Gateway Out4/1 -> Scope2/2
  Gateway Out5/1 -> Scope2/3, Scope4/1
  Relational1/1 -> Subsystem3/1(In1), Subsystem2/2(d)
  Absolute1/1 -> Relational1/1, Gateway Out18/1
  Absolute2/1 -> Gateway Out19/1, Relational3/1
  Gateway Out9/1 -> Scope4/3
  Gateway Out10/1 -> Scope4/2
  Counter/1 -> Register2/1, Gateway Out8/1, Gateway Out5/1
  Logical3/1 -> Gateway Out11/1, Gateway Out10/1, Counter/2
  [reset] -> Gateway Out9/1, Counter/1
  Delay2/1 -> Gateway Out3/1, delay_fb_latch/1
  Relational3/1 -> Subsystem1/2(d), Subsystem/1(In1), Subsystem3/2(In2)
  negedge/1(q) -> Register2/2, Subsystem2/1(lc), Subsystem1/1(lc)
  Subsystem1/1(q) -> Subsystem1/3(qb), Gateway Out2/1, Logical3/2
  Subsystem2/1(q) -> Subsystem2/3(qb), Gateway Out1/1, Logical3/1
  Subsystem3/2(or) -> negedge/1(d)
  Subsystem3/1(and) -> Gateway Out7/1
  Subsystem/1(Out1) -> Delay2/1
  Gateway Out1/1 -> Scope1/2
  Gateway Out2/1 -> Scope1/3
  Gateway Out11/1 -> Scope1/1

== system exampleModel_bus_axi_w_4ptavg/example/dsp/Cav2/c2p2_window_wf/Delay_calc2 ==
  wav : Inport
  win : Inport  Port=2
  Absolute1 : xbsIndex_r4/Absolute  precision=Full  arith_type=Unsigned  n_bits=16  bin_pt=14  quantization=Truncate  overflow=Wrap  en=off  latency=1  dbl_ovrd=off  block_type=abs
  Absolute2 : xbsIndex_r4/Absolute  precision=Full  arith_type=Unsigned  n_bits=16  bin_pt=14  quantization=Truncate  overflow=Wrap  en=off  latency=1  dbl_ovrd=off  block_type=abs
  Constant1 : xbsIndex_r4/Constant  const=0  gui_display_data_type=Fixed-point  arith_type=Signed (2's comp)  n_bits=18  bin_pt=16  preci_type=Single  exp_width=8  frac_width=24  explicit_period=off  period=1  equ=P=C  opselect=C  inp2=PCIN>>17  opr=+  inp1=P  carry=CIN  dbl_ovrd=off  block_type=constant
  Constant2 : xbsIndex_r4/Constant  const=0  gui_display_data_type=Fixed-point  arith_type=Signed (2's comp)  n_bits=2  bin_pt=0  preci_type=Single  exp_width=8  frac_width=24  explicit_period=off  period=1  equ=P=C  opselect=C  inp2=PCIN>>17  opr=+  inp1=P  carry=CIN  dbl_ovrd=off  block_type=constant
  Counter : xbsIndex_r4/Counter  cnt_type=Free Running  cnt_to=Inf  operation=Up  start_count=0  cnt_by_val=1  arith_type=Unsigned  n_bits=16  bin_pt=0  load_pin=off  rst=on  en=on  explicit_period=off  period=1  use_behavioral_HDL=off  implementation=Fabric  dbl_ovrd=off  block_type=counter
  Delay2 : xbsIndex_r4/Delay  rst=off  infoeditControl=Selection of Reset will increase slice count due to use of real FFs and instead of SRLs  en=off  latency=30  reg_retiming=off  dbl_ovrd=off  block_type=delay
  Display : Display
  Gateway Out{1..11,18..19} (13 alike) : xbsIndex_r4/Gateway Out  inherit_from_input=off  hdl_port=off  rows=1  columns=1  UseAsDAC=off  DACChannel='1'  interface=None  automatic_assignment=on  address_offset=hex2dec('00')  intf_name=''  intf_description=''  timing_constraint=None  locs_specified=off  LOCs={}  io_standard={}  block_type=gatewayout
  Logical3 : xbsIndex_r4/Logical  logical_function=XOR  inputs=2  en=off  latency=1  precision=Full  arith_type=Unsigned  n_bits=16  bin_pt=0  align_bp=on  dbl_ovrd=off  block_type=logical
  Register2 : xbsIndex_r4/Register  init=0  rst=off  en=on  dbl_ovrd=off  block_type=register
  Relational1 : xbsIndex_r4/Relational  mode=a>b  op_type=Bool  en=off  latency=1  dbl_ovrd=off  block_type=relational
  Relational3 : xbsIndex_r4/Relational  mode=a>b  op_type=Bool  en=off  latency=1  dbl_ovrd=off  block_type=relational
  Scope{1..2,4,7} (4 alike) : Scope  NumInputPorts=3
  Scope3 : Scope  NumInputPorts=2
  Subsystem : Subsystem
  Subsystem1 : Subsystem
  Subsystem2 : Subsystem
  Subsystem3 : Subsystem
  negedge : Subsystem
  delay_amt : Outport
  delay_fb_latch : Outport  Port=2
  wires:
  Gateway Out11/1 -> Scope1/1
  Gateway Out2/1 -> Scope1/3
  Gateway Out1/1 -> Scope1/2
  Subsystem/1(Out1) -> Delay2/1
  Subsystem3/1(and) -> Gateway Out7/1
  Subsystem3/2(or) -> negedge/1(d)
  Subsystem2/1(q) -> Logical3/1, Gateway Out1/1, Subsystem2/3(qb)
  Subsystem1/1(q) -> Logical3/2, Gateway Out2/1, Subsystem1/3(qb)
  negedge/1(q) -> Subsystem1/1(lc), Subsystem2/1(lc), Register2/2
  Relational3/1 -> Subsystem3/2(In2), Subsystem/1(In1), Subsystem1/2(d)
  Delay2/1 -> delay_fb_latch/1, Gateway Out3/1
  [reset] -> Counter/1, Gateway Out9/1
  Logical3/1 -> Counter/2, Gateway Out10/1, Gateway Out11/1
  Counter/1 -> Gateway Out5/1, Gateway Out8/1, Register2/1
  Gateway Out10/1 -> Scope4/2
  Gateway Out9/1 -> Scope4/3
  Absolute2/1 -> Relational3/1, Gateway Out19/1
  Absolute1/1 -> Gateway Out18/1, Relational1/1
  Relational1/1 -> Subsystem2/2(d), Subsystem3/1(In1)
  Gateway Out5/1 -> Scope4/1, Scope2/3
  Gateway Out4/1 -> Scope2/2
  Gateway Out3/1 -> Scope2/1
  Gateway Out7/1 -> Scope7/1
  Gateway Out8/1 -> Scope7/2
  Gateway Out6/1 -> Scope7/3, Display/1
  wav/1 -> Absolute1/1
  Gateway Out18/1 -> Scope3/1
  Constant1/1 -> Relational1/2
  win/1 -> Absolute2/1
  Constant2/1 -> Relational3/2
  Gateway Out19/1 -> Scope3/2
  Register2/1 -> delay_amt/1, Gateway Out6/1, Gateway Out4/1

== system exampleModel_bus_axi_w_4ptavg/example/dsp/Cav1/Subsystem/freq_err/delta_phi ==
  note: d(scaled_phi)
  note: calculating delta phi
  note: 3.14
  phase : Inport
  window : Inport  Port=2
  reset : Inport  Port=3
  AddSub3 : xbsIndex_r4/AddSub  mode=Subtraction  use_carryin=off  use_carryout=off  en=on  latency=1  precision=User Defined  arith_type="Signed  (2's comp)"  n_bits=32  bin_pt=30  quantization=Truncate  overflow=Saturate  use_behavioral_HDL=off  hw_selection=Fabric  pipelined=off  dbl_ovrd=off  block_type=addsub
  Constant : xbsIndex_r4/Constant  const=0  gui_display_data_type=Fixed-point  arith_type=Signed (2's comp)  n_bits=1  bin_pt=0  preci_type=Single  exp_width=8  frac_width=24  explicit_period=off  period=1  equ=P=C  opselect=C  inp2=PCIN>>17  opr=+  inp1=P  carry=CIN  dbl_ovrd=off  block_type=constant
  Constant1 : xbsIndex_r4/Constant  const=0  gui_display_data_type=Fixed-point  arith_type=Signed (2's comp)  n_bits=1  bin_pt=0  preci_type=Single  exp_width=8  frac_width=24  explicit_period=off  period=1  equ=P=C  opselect=C  inp2=PCIN>>17  opr=+  inp1=P  carry=CIN  dbl_ovrd=off  block_type=constant
  Constant4 : xbsIndex_r4/Constant  const=pi  gui_display_data_type=Fixed-point  arith_type=Signed (2's comp)  n_bits=18  bin_pt=15  preci_type=Single  exp_width=8  frac_width=24  explicit_period=off  period=1  equ=P=C  opselect=C  inp2=PCIN>>17  opr=+  inp1=P  carry=CIN  dbl_ovrd=off  block_type=constant
  Convert1 : xbsIndex_r4/Convert  gui_display_data_type=Boolean  arith_type=Boolean  n_bits=16  bin_pt=14  float_type=Single  exp_bits=8  fraction_bits=24  quantization=Truncate  overflow=Wrap  en=off  latency=1  pipeline=off  dbl_ovrd=off  block_type=convert
  Delay2 : xbsIndex_r4/Delay  rst=off  infoeditControl=Selection of Reset will increase slice count due to use of real FFs and instead of SRLs  en=off  latency=2  reg_retiming=off  dbl_ovrd=off  block_type=delay
  Display{,1..2,5} (4 alike) : Display
  Gateway Out{3,27..29} (4 alike) : xbsIndex_r4/Gateway Out  inherit_from_input=off  hdl_port=on  rows=1  columns=1  UseAsDAC=off  DACChannel='1'  interface=None  automatic_assignment=on  address_offset=hex2dec('00')  intf_name=''  intf_description=''  timing_constraint=None  locs_specified=off  LOCs={}  io_standard={}  block_type=gatewayout
  Inverter : xbsIndex_r4/Inverter  en=off  latency=1  dbl_ovrd=off  block_type=inv
  Logical : xbsIndex_r4/Logical  logical_function=AND  inputs=2  en=off  latency=1  precision=User Defined  arith_type=Boolean  n_bits=1  bin_pt=0  align_bp=on  dbl_ovrd=off  block_type=logical
  Mult1 : xbsIndex_r4/Mult  precision=User Defined  arith_type="Signed  (2's comp)"  n_bits=32  bin_pt=30  quantization=Truncate  overflow=Saturate  en=off  latency=3  use_behavioral_HDL=off  opt=Speed  use_embedded=on  optimum_pipeline=off  pipeline=on  dbl_ovrd=off  use_rpm=on  placement_style=Triangular  block_type=mult
  Relational : xbsIndex_r4/Relational  mode=a!=b  op_type=Bool  en=off  latency=1  dbl_ovrd=off  block_type=relational
  Relational1 : xbsIndex_r4/Relational  mode=a!=b  op_type=Bool  en=off  latency=1  dbl_ovrd=off  block_type=relational
  hi_bits : Scope  NumInputPorts=4
  phase_latching : Subsystem
  d_phi : Outport
  val_latched : Outport  Port=2
  wires:
  reset/1 -> phase_latching/3(reset)
  Inverter/1 -> Delay2/1
  Constant4/1 -> Mult1/2
  Gateway Out3/1 -> hi_bits/4, Display5/1
  Delay2/1 -> AddSub3/3
  Gateway Out29/1 -> hi_bits/1, Display/1
  Mult1/1 -> d_phi/1, Gateway Out3/1
  phase/1 -> phase_latching/1(phase)
  AddSub3/1 -> Mult1/1, Gateway Out27/1
  Gateway Out28/1 -> hi_bits/2, Display1/1
  Gateway Out27/1 -> hi_bits/3, Display2/1
  Convert1/1 -> Inverter/1
  window/1 -> Convert1/1, phase_latching/2(window)
  phase_latching/1(Stop_value) -> AddSub3/1, Relational/1, Gateway Out29/1
  Constant/1 -> Relational/2
  Constant1/1 -> Relational1/2
  phase_latching/2(Start_value) -> Relational1/1, Gateway Out28/1, AddSub3/2
  Relational/1 -> Logical/1
  Relational1/1 -> Logical/2
  Logical/1 -> val_latched/1

== system exampleModel_bus_axi_w_4ptavg/example/dsp/Cav1/Subsystem/freq_err/delta_t ==
  note: (2*pi)/(Fsig)
  window : Inport
  reset : Inport  Port=2
  Constant5 : xbsIndex_r4/Constant  const=(2*pi)/(Fsig)  gui_display_data_type=Fixed-point  arith_type=Unsigned  n_bits=32  bin_pt=32  preci_type=Single  exp_width=8  frac_width=24  explicit_period=off  period=1  equ=P=C  opselect=C  inp2=PCIN>>17  opr=+  inp1=P  carry=CIN  dbl_ovrd=off  block_type=constant
  Convert1 : xbsIndex_r4/Convert  gui_display_data_type=Boolean  arith_type=Boolean  n_bits=16  bin_pt=14  float_type=Single  exp_bits=8  fraction_bits=24  quantization=Truncate  overflow=Wrap  en=off  latency=1  pipeline=off  dbl_ovrd=off  block_type=convert
  Counter2 : xbsIndex_r4/Counter  cnt_type=Free Running  cnt_to=Inf  operation=Up  start_count=0  cnt_by_val=1  arith_type=Unsigned  n_bits=10  bin_pt=0  load_pin=off  rst=on  en=on  explicit_period=on  period=1/(17e6)  use_behavioral_HDL=off  implementation=Fabric  dbl_ovrd=off  block_type=counter
  Display3 : Display
  Display4 : Display
  Gateway Out1 : xbsIndex_r4/Gateway Out  inherit_from_input=off  hdl_port=on  rows=1  columns=1  UseAsDAC=off  DACChannel='1'  interface=None  automatic_assignment=on  address_offset=hex2dec('00')  intf_name=''  intf_description=''  timing_constraint=None  locs_specified=off  LOCs={}  io_standard={}  block_type=gatewayout
  Gateway Out2 : xbsIndex_r4/Gateway Out  inherit_from_input=off  hdl_port=on  rows=1  columns=1  UseAsDAC=off  DACChannel='1'  interface=None  automatic_assignment=on  address_offset=hex2dec('00')  intf_name=''  intf_description=''  timing_constraint=None  locs_specified=off  LOCs={}  io_standard={}  block_type=gatewayout
  Inverter : xbsIndex_r4/Inverter  en=off  latency=1  dbl_ovrd=off  block_type=inv
  Mult : xbsIndex_r4/Mult  precision=User Defined  arith_type="Signed  (2's comp)"  n_bits=32  bin_pt=32  quantization=Truncate  overflow=Saturate  en=off  latency=3  use_behavioral_HDL=off  opt=Speed  use_embedded=on  optimum_pipeline=off  pipeline=on  dbl_ovrd=off  use_rpm=on  placement_style=Triangular  block_type=mult
  Register2 : xbsIndex_r4/Register  init=0  rst=on  en=on  dbl_ovrd=off  block_type=register
  dt : Outport
  wires:
  reset/1 -> Register2/2, Counter2/1
  Register2/1 -> Mult/1, Gateway Out2/1
  Gateway Out2/1 -> Display4/1
  Counter2/1 -> Register2/1
  Inverter/1 -> Register2/3
  Convert1/1 -> Inverter/1, Counter2/2
  Constant5/1 -> Mult/2
  Mult/1 -> dt/1, Gateway Out1/1
  window/1 -> Convert1/1
  Gateway Out1/1 -> Display3/1

== system exampleModel_bus_axi_w_4ptavg/example/dsp/Cav1/c1p1_freq_err_module/freq_err1/Subsystem ==
  In1 : Inport
  In2 : Inport  Port=2
  AddSub : xbsIndex_r4/AddSub  mode=Addition  use_carryin=off  use_carryout=off  en=on  latency=1  precision=User Defined  arith_type="Signed  (2's comp)"  n_bits=64  bin_pt=32  quantization=Truncate  overflow=Saturate  use_behavioral_HDL=off  hw_selection=Fabric  pipelined=off  dbl_ovrd=off  block_type=addsub
  Constant1 : xbsIndex_r4/Constant  const=-Fsig  gui_display_data_type=Fixed-point  arith_type=Signed (2's comp)  n_bits=26  bin_pt=0  preci_type=Single  exp_width=8  frac_width=24  explicit_period=off  period=1  equ=P=C  opselect=C  inp2=PCIN>>17  opr=+  inp1=P  carry=CIN  dbl_ovrd=off  block_type=constant
  Convert1 : xbsIndex_r4/Convert  gui_display_data_type=Fixed-point  arith_type="Signed  (2's comp)"  n_bits=32  bin_pt=32  float_type=Single  exp_bits=8  fraction_bits=24  quantization=Truncate  overflow=Saturate  en=off  latency=1  pipeline=off  dbl_ovrd=off  block_type=convert
  Delay3 : xbsIndex_r4/Delay  rst=off  infoeditControl=Selection of Reset will increase slice count due to use of real FFs and instead of SRLs  en=off  latency=10  reg_retiming=off  dbl_ovrd=off  block_type=delay
  Delay4 : xbsIndex_r4/Delay  rst=off  infoeditControl=Selection of Reset will increase slice count due to use of real FFs and instead of SRLs  en=off  latency=1  reg_retiming=off  dbl_ovrd=off  block_type=delay
  Delay5 : xbsIndex_r4/Delay  rst=off  infoeditControl=Selection of Reset will increase slice count due to use of real FFs and instead of SRLs  en=off  latency=1  reg_retiming=off  dbl_ovrd=off  block_type=delay
  Display1 : Display
  Divide2 : xbsIndex_r4/Divide  flow_control=NonBlocking  axi_optimize_goal=Resources  algorithm_type=Radix2  infoedit1=Specify output fraction-width for Fixed-point division.  fractional_width=33  infoedit2=Specify latency for Floating-point division.  latency=1  rate=1  has_a_tlast=off  has_a_tuser=off  has_b_tlast=off  has_b_tuser=off  en=off  has_result_tready=off  result_tlast_behv=Pass_A_TLAST  has_underflow=off  has_overflow=off  has_invalid_op=off  has_divide_by_zero=off  fpo_op_type=mergeddivide  block_type=divide
      settings: infoedit=Blocking: Wait for data on all inputs, allow back-pressure.<br>NonBlocking: operate every cycle in which all inputs are valid, no back-pressure.
  Down Sample1 : xbsIndex_r4/Down Sample  sample_ratio=12  sample_phase="Last Value of Frame  (most efficient)"  en=off  rst=off  latency=1  dbl_ovrd=off  block_type=dsamp
  Down Sample8 : xbsIndex_r4/Down Sample  sample_ratio=12  sample_phase="Last Value of Frame  (most efficient)"  en=off  rst=off  latency=1  dbl_ovrd=off  block_type=dsamp
  Gateway Out{5..7,9} (4 alike) : xbsIndex_r4/Gateway Out  inherit_from_input=off  hdl_port=on  rows=1  columns=1  UseAsDAC=off  DACChannel='1'  interface=None  automatic_assignment=on  address_offset=hex2dec('00')  intf_name=''  intf_description=''  timing_constraint=None  locs_specified=off  LOCs={}  io_standard={}  block_type=gatewayout
  Inverter : xbsIndex_r4/Inverter  en=off  latency=1  dbl_ovrd=off  block_type=inv
  Logical1 : xbsIndex_r4/Logical  logical_function=AND  inputs=2  en=off  latency=1  precision=User Defined  arith_type=Boolean  n_bits=1  bin_pt=0  align_bp=on  dbl_ovrd=off  block_type=logical
  Register : xbsIndex_r4/Register  init=0  rst=on  en=on  dbl_ovrd=off  block_type=register
  Scope3 : Scope  NumInputPorts=3
  Scope4 : Scope  NumInputPorts=3
  tag scope: testb=global
  wires:
  Delay3/1 -> Logical1/2, Inverter/1
  Logical1/1 -> Gateway Out6/1, Delay4/1, Delay5/1, Register/3
  Constant1/1 -> Divide2/2
  Inverter/1 -> Logical1/1
  Divide2/1 -> Down Sample1/1
  Register/1 -> AddSub/1, Gateway Out5/1
  Gateway Out5/1 -> Scope3/2
  In2/1 -> Down Sample8/1
  Convert1/1 -> [testb]
  Down Sample8/1 -> Register/1
  Delay5/1 -> Register/2
  Delay4/1 -> AddSub/3
  Gateway Out6/1 -> Scope3/3
  In1/1 -> Delay3/1
  AddSub/1 -> AddSub/2, Gateway Out7/1, Divide2/1, Gateway Out9/1
  Down Sample1/1 -> Convert1/1
  Gateway Out7/1 -> Scope3/1, Display1/1
  Gateway Out9/1 -> Scope4/1
